simulink model "Simulation"  (R2019b)
settings: Solver=VariableStepAuto  StartTime=0.0  StopTime=T_total  RelTol=1e-3
undefined symbols (not defined in the file): C, DiscIntNeverNeededParam, G, Gex, Seed, Tsim
libraries: dspsrcs4 x5
settings Model: SimulationMode=accelerator  Creator=Downstream  LastModifiedBy=Downstream

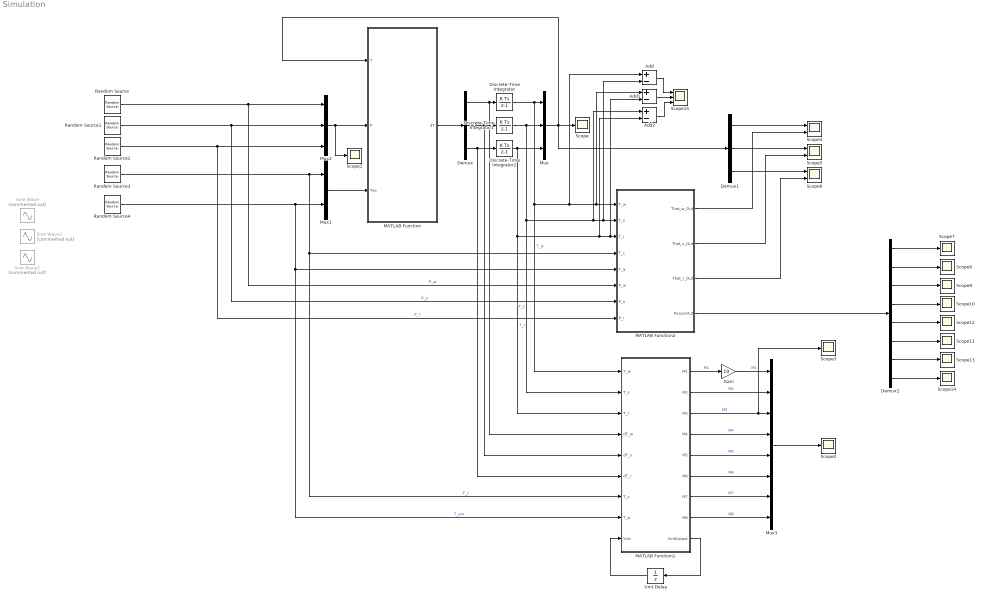
== system Simulation ==
  Add : Sum  Inputs=+-
  Add1 : Sum  Inputs=+-
  Add2 : Sum  Inputs=+-
  Demux : Demux  Outputs=3
  Demux1 : Demux  Outputs=3
  Demux2 : Demux  Outputs=8
  Discrete-Time Integrator : DiscreteIntegrator  InitialCondition=20  SampleTime=-1  ICPrevOutput=DiscIntNeverNeededParam  ICPrevScaledInput=DiscIntNeverNeededParam
  Discrete-Time Integrator1 : DiscreteIntegrator  InitialCondition=20  SampleTime=-1  ICPrevOutput=DiscIntNeverNeededParam  ICPrevScaledInput=DiscIntNeverNeededParam
  Discrete-Time Integrator2 : DiscreteIntegrator  InitialCondition=20  SampleTime=-1  ICPrevOutput=DiscIntNeverNeededParam  ICPrevScaledInput=DiscIntNeverNeededParam
  Gain : Gain  Gain=10
  MATLAB Function : MATLAB Function  TreatAsAtomicUnit=on  SystemSampleTime=Tsim
  MATLAB Function1 : MATLAB Function  TreatAsAtomicUnit=on
  MATLAB Function2 : MATLAB Function  TreatAsAtomicUnit=on
  Mux : Mux  Inputs=3
  Mux1 : Mux  Inputs=2
  Mux2 : Mux  Inputs=3
  Mux3 : Mux  Inputs=8
  Random Source : dspsrcs4/Random Source  SrcType=Uniform  NormMethod=Ziggurat  CltLength=12  MinVal=0  MaxVal=1000  MeanVal=0  VarVal=1  RepMode=Specify seed  rawSeed=Seed(1)  IsInherit=off  SampMode=Discrete  SampTime=Ts_p  SampFrame=1  DataType=Double  OutComplex=Real  OutputFrames=off
  Random Source1 : dspsrcs4/Random Source  SrcType=Uniform  NormMethod=Ziggurat  CltLength=12  MinVal=0  MaxVal=1000  MeanVal=0  VarVal=1  RepMode=Specify seed  rawSeed=Seed(2)  IsInherit=off  SampMode=Discrete  SampTime=Ts_p  SampFrame=1  DataType=Double  OutComplex=Real  OutputFrames=off
  Random Source2 : dspsrcs4/Random Source  SrcType=Uniform  NormMethod=Ziggurat  CltLength=12  MinVal=0  MaxVal=1000  MeanVal=0  VarVal=1  RepMode=Specify seed  rawSeed=Seed(3)  IsInherit=off  SampMode=Discrete  SampTime=Ts_p  SampFrame=1  DataType=Double  OutComplex=Real  OutputFrames=off
  Random Source3 : dspsrcs4/Random Source  SrcType=Uniform  NormMethod=Ziggurat  CltLength=12  MinVal=20  MaxVal=50  MeanVal=0  VarVal=1  RepMode=Specify seed  rawSeed=Seed(4)  IsInherit=off  SampMode=Discrete  SampTime=Ts_c  SampFrame=1  DataType=Double  OutComplex=Real  OutputFrames=off
  Random Source4 : dspsrcs4/Random Source  SrcType=Uniform  NormMethod=Ziggurat  CltLength=12  MinVal=20  MaxVal=50  MeanVal=0  VarVal=1  RepMode=Specify seed  rawSeed=Seed(5)  IsInherit=off  SampMode=Discrete  SampTime=Ts_am  SampFrame=1  DataType=Double  OutComplex=Real  OutputFrames=off
  Scope{,1..3,7..14} (12 alike) : Scope
  Scope15 : Scope  NumInputPorts=3
  Scope4 : Scope  NumInputPorts=2
  Scope5 : Scope  NumInputPorts=2
  Scope6 : Scope  NumInputPorts=2
  Sine Wave : Sin  Commented=on  Amplitude=1000  Bias=1000  Frequency=0.001*2*pi  SampleTime=0
  Sine Wave1 : Sin  Commented=on  Amplitude=1000  Bias=2000  Frequency=0.002*2*pi  SampleTime=0
  Sine Wave2 : Sin  Commented=on  Amplitude=500  Bias=2000  Frequency=0.003*2*pi  SampleTime=0
  Unit Delay : UnitDelay  SampleTime=-1  HasFrameUpgradeWarning=on
  wires:
  MATLAB Function/1(dT) -> Demux/1
  Mux/1 -> Scope/1, MATLAB Function/1(T), Demux1/1
  Mux2/1 -> Scope1/1, MATLAB Function/2(P)
  Mux1/1 -> MATLAB Function/3(Tex)
  Random Source/1 -> Mux2/1, MATLAB Function2/6(P_w)  "P_w"
  Random Source1/1 -> Mux2/2, MATLAB Function2/7(P_s)  "P_s"
  Random Source2/1 -> Mux2/3, MATLAB Function2/8(P_r)  "P_r"
  MATLAB Function1/9(VintOutput) -> Unit Delay/1
  Unit Delay/1 -> MATLAB Function1/9(Vint)
  MATLAB Function1/5(M5) -> Mux3/5  "M5"
  MATLAB Function1/4(M4) -> Mux3/4  "M4"
  MATLAB Function1/3(M3) -> Scope3/1, Mux3/3  "M3"
  MATLAB Function1/2(M2) -> Mux3/2  "M2"
  MATLAB Function1/1(M1) -> Gain/1  "M1"
  MATLAB Function1/6(M6) -> Mux3/6  "M6"
  MATLAB Function1/7(M7) -> Mux3/7  "M7"
  MATLAB Function1/8(M8) -> Mux3/8  "M8"
  Mux3/1 -> Scope2/1
  Gain/1 -> Mux3/1  "M1"
  Demux1/1 -> Scope4/1
  MATLAB Function2/1(That_w_Out) -> Scope4/2
  Demux1/2 -> Scope5/1
  Demux1/3 -> Scope6/1
  MATLAB Function2/2(That_s_Out) -> Scope5/2
  MATLAB Function2/3(That_r_Out) -> Scope6/2
  MATLAB Function2/4(ParamOut) -> Demux2/1
  Demux2/1 -> Scope7/1
  Demux2/2 -> Scope8/1
  Demux2/3 -> Scope9/1
  Demux2/4 -> Scope10/1
  Demux2/5 -> Scope12/1
  Demux2/6 -> Scope11/1
  Demux2/7 -> Scope13/1
  Demux2/8 -> Scope14/1
  Add/1 -> Scope15/1
  Add1/1 -> Scope15/2
  Add2/1 -> Scope15/3
  Random Source4/1 -> MATLAB Function2/5(T_a), MATLAB Function1/8(T_a), Mux1/2  "T_am"
  Random Source3/1 -> MATLAB Function2/4(T_c), MATLAB Function1/7(T_c), Mux1/1  "T_c"
  Discrete-Time Integrator1/1 -> Add2/1, Add/2, MATLAB Function2/2(T_s), MATLAB Function1/2(T_s), Mux/2  "T_s"
  Discrete-Time Integrator2/1 -> Add2/2, Add1/2, MATLAB Function2/3(T_r), MATLAB Function1/3(T_r), Mux/3  "T_r"
  Discrete-Time Integrator/1 -> Add/1, Add1/1, MATLAB Function2/1(T_w), MATLAB Function1/1(T_w), Mux/1  "T_w"
  Demux/3 -> MATLAB Function1/6(dT_r), Discrete-Time Integrator2/1
  Demux/2 -> MATLAB Function1/5(dT_s), Discrete-Time Integrator1/1
  Demux/1 -> MATLAB Function1/4(dT_w), Discrete-Time Integrator/1

== matlab function Simulation/MATLAB Function1 ==
  data: T_w input; M1 output; T_s input; T_r input; dT_w input; dT_s input; dT_r input; M2 output; M3 output; M4 output; M5 output; M6 output; M7 output; M8 output; T_c input; T_a input; Vint input; VintOutput output
function [M1,M2,M3,M4,M5,M6,M7,M8,VintOutput] = PECondition(T_w,T_s,T_r,dT_w,dT_s,dT_r,T_c,T_a,Vint)
Tsim = 0.1;
Psi = [T_s - T_w, T_r - T_w, 0        , 0        , 0        , -dT_w, 0    , 0    ;
       T_w - T_s, 0        , T_r - T_s, T_c - T_s, 0        , 0    , -dT_s, 0    ;
       0        , T_w - T_r, T_s - T_r, 0        , T_a - T_r, 0    , 0    , -dT_r;];
V = Psi' * Psi;
VintOutput = Vint + V .* Tsim;
M1 = det(V(1:1,1:1));
M2 = det(V(1:2,1:2));
M3 = det(V(1:3,1:3));
M4 = det(V(1:4,1:4));
M5 = det(V(1:5,1:5));
M6 = det(V(1:6,1:6));
M7 = det(V(1:7,1:7));
M8 = det(V(1:8,1:8));

% y = u;

== matlab function Simulation/MATLAB Function ==
  data: T input; dT output; P input; Tex input; Gex parameter; G parameter; C parameter
function dT = LPTN(T,P,Tex,Gex, G, C)
Temp = -G * T + Gex * Tex + P;
dT = C^-1 * Temp;

== matlab function Simulation/MATLAB Function2 ==
  data: T_w input; That_w_Out output; T_s input; T_r input; T_c input; T_a input; P_w input; P_s input; P_r input; That_s_Out output; That_r_Out output; ParamOut output
function [That_w_Out,That_s_Out,That_r_Out,ParamOut] = MRAS(T_w,T_s,T_r,T_c,T_a,P_w,P_s,P_r)
persistent T_hat Ghat_c2s Ghat_w2r Ghat_r2a Chat_s Chat_w Chat_r Ghat_s2w Ghat_s2r
Tsim = 0.1;
if isempty(T_hat)
    T_hat = [20;20;20;];
    Ghat_c2s = 110; Ghat_w2r = 29; Ghat_r2a = 9; Chat_s = 5000; Chat_w = 2500; Chat_r = 8000;
    Ghat_s2w = 83;  Ghat_s2r = 40;
end
P = [P_w,P_s,P_r]';
T = [T_w,T_s,T_r]';
Tex = [T_c, T_a]';

T_tilde = T_hat - T;

Ghat = [Ghat_s2w + Ghat_w2r, -Ghat_s2w                      ,   -Ghat_w2r                     ;
        -Ghat_s2w          ,  Ghat_s2w + Ghat_c2s + Ghat_s2r,   -Ghat_s2r                     ;
        -Ghat_w2r          , -Ghat_s2r                      ,   Ghat_r2a + Ghat_s2r + Ghat_w2r;];
Gexhat = [0 Ghat_c2s 0    ;
          0 0     Ghat_r2a;]';
Chat = diag([Chat_w Chat_s Chat_r]);

Temp = -Ghat * T_hat + Gexhat * Tex + P;
Temp = (Chat^-1) * Temp;

Psi = [T_hat(2) - T_hat(1), T_hat(3) - T_hat(1), 0                  , 0             , 0             , -Temp(1), 0       , 0       ;
       T_hat(1) - T_hat(2), 0                  , T_hat(3) - T_hat(2), T_c - T_hat(2), 0             , 0       , -Temp(2), 0       ;
       0                  , T_hat(1) - T_hat(3), T_hat(2) - T_hat(3), 0             , T_a - T_hat(3), 0       , 0       , -Temp(3);];
dTheta = -0.1 .* (T_tilde' * Psi)' .* Tsim;
Ghat_s2w = Ghat_s2w + dTheta(1);
Ghat_w2r = Ghat_w2r + dTheta(2);
Ghat_s2r = Ghat_s2r + dTheta(3);
Ghat_c2s = Ghat_c2s + dTheta(4);
Ghat_r2a = Ghat_r2a + dTheta(5);
Chat_w = Chat_w + dTheta(6);
Chat_s = Chat_s + dTheta(7);
Chat_r = Chat_r + dTheta(8);

Chat_s = 5000; 
Chat_w = 2500; 
Chat_r = 8000;
Ghat_c2s = 111.1111;
Ghat_r2a = 8.33333;
   

T_hat = T_hat + Temp .* Tsim;
That_w_Out = T_hat(1);
That_s_Out = T_hat(2);
That_r_Out = T_hat(3);


ParamOut = [Ghat_s2w,Ghat_w2r,Ghat_s2r,Ghat_c2s,Ghat_r2a,Chat_w,Chat_s,Chat_r];
